simulink library "my_library"  (Simulink 4.00)
undefined symbols (not defined in the file or in its folder): get
libraries: dspsigops x4, dspddes3 x3, dsplibv4 x2, dsparch3 x1, dspbuff3 x1, dspspect3 x1, dspstat3 x1, dspsnks3 x1
settings Model: LastModifiedBy=Administrator

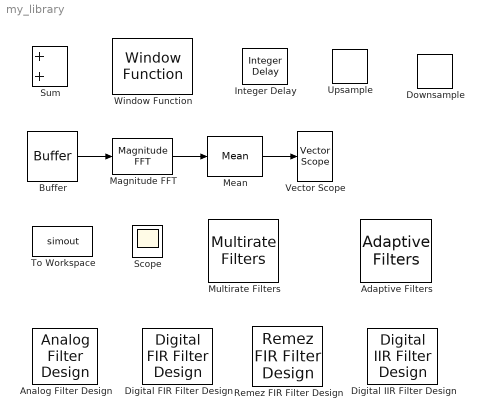
== system my_library ==
  Adaptive Filters : dsplibv4/Filtering/Adaptive Filters
  Analog Filter Design : dsparch3/Analog Filter Design  method=Butterworth  filttype=Lowpass  N=8  Wlo=30  Whi=80  Rp=2  Rs=40
  Buffer : dspbuff3/Buffer  N=64  V=0  ic=0
  Digital FIR Filter Design : dspddes3/Digital FIR Filter Design  filttype=Lowpass  N=22  Wlo=0.4  Whi=0.6  W0=[.2 .5 .8]  g0=1  W1=[0 .2 .3 .6 .8 1]  gains=[1 .5 0 0 1 .5]  wintype=Hamming  Rs=10  Kbeta=5
  Digital IIR Filter Design : dspddes3/Digital IIR Filter Design  method=Butterworth  filttype=Lowpass  N=4  Wlo=0.4  Whi=0.6  Rp=2  Rs=20
  Downsample : dspsigops/Downsample  N=2  phase=0  ic=0  smode=Allow multirate  fmode=Maintain input frame size
  Integer Delay : dspsigops/Integer Delay  delay=1  ic=0
  Magnitude FFT : dspspect3/Magnitude FFT  fftLenInherit=off  fftsize=256
  Mean : dspstat3/Mean  run=on  reset_popup=None
  Multirate Filters : dsplibv4/Filtering/Multirate Filters
  Remez FIR Filter Design : dspddes3/Remez FIR Filter Design  filttype=Multiband  F=[0 0.4 0.5 1]  A=[1 1 0 0]  W=[1 1]  N=23
  Scope : Scope
      settings: TimeRange=auto  YMin=-5  YMax=5  SaveToWorkspace=off  SaveName=ScopeData  LimitDataPoints=on  MaxDataPoints=5000
  Sum : Sum  Inputs=++  SaturateOnIntegerOverflow=on
  To Workspace : ToWorkspace  VariableName=simout  SampleTime=-1  SaveFormat=Structure
  Upsample : dspsigops/Upsample  N=3  phase=0  ic=0  mode=Maintain input frame size
  Vector Scope : dspsnks3/Vector Scope  ScopeProperties=off  Domain=Frequency  HorizSpan=1  DisplayProperties=off  AxisGrid=on  Memory=off  FrameNumber=on  AxisLegend=off  AxisZoom=off  OpenScopeAtSimStart=on  OpenScopeImmediately=off  FigPos=get(0,'defaultfigureposition')  AxisProperties=on  XUnits=Hertz  XRange=[0...Fs/2]  InheritXIncr=on  XIncr=1  XLabel=Time  YUnits=dB  YLabel=Amplitude  LineProperties=off
      settings: YMin=-10  YMax=10
  Window Function : dspsigops/Window Function  winmode=Apply window to input  wintype=Hamming  N=64  Rs=50  beta=10  winsamp=Symmetric  UserWindow=hamming  OptParams=off  UserParams={1.0}
  wires:
  Magnitude FFT/1 -> Mean/1
  Buffer/1 -> Magnitude FFT/1
  Mean/1 -> Vector Scope/1
